simulink model "functional_architecture"  (R2019b)
settings: Solver=VariableStepAuto  StartTime=0.0  StopTime=10.0  RelTol=1e-3
settings Model: Creator=nicol  LastModifiedBy=nicol

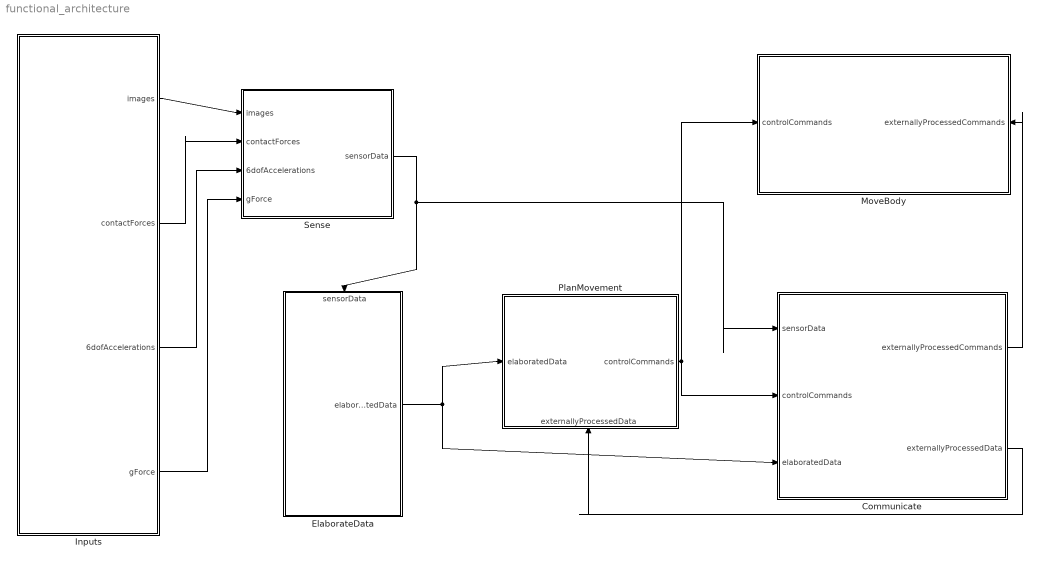
== system functional_architecture ==
  Communicate : Subsystem
      settings: PortSchema="{\"entries\":[{\"content\":{\"headerSize\":26,\"margin\":15,\"minimumSpacing\":25,\"sides\":[{\"content\":{\"connectorIds\":[\"In1\",\"In2\",\"In3\"]},\"type\":\"ConnectorPlacement.EquallySpacedRectSide\",\"uuid\":\"1a5b96a6-6b68-4a44-94ba-f4f30127e72c\"},{\"content\":{\"connectorIds\":[\"Out1\",\"Out2\"],\"side\":\"RIGHT\"},\"type\":\"ConnectorPlacement.EquallySpacedRectSide\",\"uuid\":\"6795999a-37c2-4f74-9b2a-5ff47da3b2b8\"},{\"content\":{\"connectorIds\":[],\"side\":\"TOP\"},\"type\":\"ConnectorPlacement.EquallySpacedRectSide\",\"uuid\":\"71a167ad-2262-404f-8290-656c4c9ef881\"},{\"content\":{\"connectorIds\":[],\"side\":\"BOTTOM\"},\"type\":\"ConnectorPlacement.EquallySpacedRectSide\",\"uuid\":\"bd9bb314-13dd-4e4e-ba5b-ba97c08285c9\"}]},\"type\":\"ConnectorPlacement.EquallySpacedConnector\",\"uuid\":\"f8e426a6-4f1d-49ba-8aa9-835f0600076a\"}],\"packageUris\":[\"http://schema.mathworks.com/mf0/Connector/19700101\"],\"version\":\"1.0\"}"
  ElaborateData : Subsystem
      settings: PortSchema="{\"entries\":[{\"content\":{\"headerSize\":26,\"margin\":15,\"minimumSpacing\":25,\"sides\":[{\"content\":{\"connectorIds\":[]},\"type\":\"ConnectorPlacement.EquallySpacedRectSide\",\"uuid\":\"1a5b96a6-6b68-4a44-94ba-f4f30127e72c\"},{\"content\":{\"connectorIds\":[\"Out1\"],\"side\":\"RIGHT\"},\"type\":\"ConnectorPlacement.EquallySpacedRectSide\",\"uuid\":\"6795999a-37c2-4f74-9b2a-5ff47da3b2b8\"},{\"content\":{\"connectorIds\":[\"In1\"],\"side\":\"TOP\"},\"type\":\"ConnectorPlacement.EquallySpacedRectSide\",\"uuid\":\"71a167ad-2262-404f-8290-656c4c9ef881\"},{\"content\":{\"connectorIds\":[],\"side\":\"BOTTOM\"},\"type\":\"ConnectorPlacement.EquallySpacedRectSide\",\"uuid\":\"ec60985d-ce8e-4674-8cef-feb300bcbcea\"}]},\"type\":\"ConnectorPlacement.EquallySpacedConnector\",\"uuid\":\"f8e426a6-4f1d-49ba-8aa9-835f0600076a\"}],\"packageUris\":[\"http://schema.mathworks.com/mf0/Connector/19700101\"],\"version\":\"1.0\"}"
  Inputs : Subsystem
      settings: PortSchema="{\"entries\":[{\"content\":{\"headerSize\":26,\"margin\":15,\"minimumSpacing\":25,\"sides\":[{\"content\":{\"connectorIds\":[]},\"type\":\"ConnectorPlacement.EquallySpacedRectSide\",\"uuid\":\"1a5b96a6-6b68-4a44-94ba-f4f30127e72c\"},{\"content\":{\"connectorIds\":[\"Out1\",\"Out2\",\"Out3\",\"Out4\"],\"side\":\"RIGHT\"},\"type\":\"ConnectorPlacement.EquallySpacedRectSide\",\"uuid\":\"6795999a-37c2-4f74-9b2a-5ff47da3b2b8\"},{\"content\":{\"connectorIds\":[],\"side\":\"TOP\"},\"type\":\"ConnectorPlacement.EquallySpacedRectSide\",\"uuid\":\"71a167ad-2262-404f-8290-656c4c9ef881\"}]},\"type\":\"ConnectorPlacement.EquallySpacedConnector\",\"uuid\":\"f8e426a6-4f1d-49ba-8aa9-835f0600076a\"}],\"packageUris\":[\"http://schema.mathworks.com/mf0/Connector/19700101\"],\"version\":\"1.0\"}"
  MoveBody : Subsystem
      settings: PortSchema="{\"entries\":[{\"content\":{\"headerSize\":26,\"margin\":15,\"minimumSpacing\":25,\"sides\":[{\"content\":{\"connectorIds\":[\"In2\"]},\"type\":\"ConnectorPlacement.EquallySpacedRectSide\",\"uuid\":\"1a5b96a6-6b68-4a44-94ba-f4f30127e72c\"},{\"content\":{\"connectorIds\":[\"In1\"],\"side\":\"RIGHT\"},\"type\":\"ConnectorPlacement.EquallySpacedRectSide\",\"uuid\":\"6795999a-37c2-4f74-9b2a-5ff47da3b2b8\"},{\"content\":{\"connectorIds\":[],\"side\":\"TOP\"},\"type\":\"ConnectorPlacement.EquallySpacedRectSide\",\"uuid\":\"71a167ad-2262-404f-8290-656c4c9ef881\"},{\"content\":{\"connectorIds\":[],\"side\":\"BOTTOM\"},\"type\":\"ConnectorPlacement.EquallySpacedRectSide\",\"uuid\":\"ac9fe140-66f2-4256-968c-2b10322560fd\"}]},\"type\":\"ConnectorPlacement.EquallySpacedConnector\",\"uuid\":\"f8e426a6-4f1d-49ba-8aa9-835f0600076a\"}],\"packageUris\":[\"http://schema.mathworks.com/mf0/Connector/19700101\"],\"version\":\"1.0\"}"
  PlanMovement : Subsystem
      settings: PortSchema="{\"entries\":[{\"content\":{\"headerSize\":26,\"margin\":15,\"minimumSpacing\":25,\"sides\":[{\"content\":{\"connectorIds\":[\"In1\"]},\"type\":\"ConnectorPlacement.EquallySpacedRectSide\",\"uuid\":\"1a5b96a6-6b68-4a44-94ba-f4f30127e72c\"},{\"content\":{\"connectorIds\":[\"Out1\"],\"side\":\"RIGHT\"},\"type\":\"ConnectorPlacement.EquallySpacedRectSide\",\"uuid\":\"6795999a-37c2-4f74-9b2a-5ff47da3b2b8\"},{\"content\":{\"connectorIds\":[],\"side\":\"TOP\"},\"type\":\"ConnectorPlacement.EquallySpacedRectSide\",\"uuid\":\"71a167ad-2262-404f-8290-656c4c9ef881\"},{\"content\":{\"connectorIds\":[\"In2\"],\"side\":\"BOTTOM\"},\"type\":\"ConnectorPlacement.EquallySpacedRectSide\",\"uuid\":\"7978899b-6d5b-49fc-849e-56f3629990a5\"}]},\"type\":\"ConnectorPlacement.EquallySpacedConnector\",\"uuid\":\"f8e426a6-4f1d-49ba-8aa9-835f0600076a\"}],\"packageUris\":[\"http://schema.mathworks.com/mf0/Connector/19700101\"],\"version\":\"1.0\"}"
  Sense : Subsystem
      settings: PortSchema="{\"entries\":[{\"content\":{\"headerSize\":26,\"margin\":15,\"minimumSpacing\":25,\"sides\":[{\"content\":{\"connectorIds\":[\"In1\",\"In2\",\"In3\",\"In4\"]},\"type\":\"ConnectorPlacement.EquallySpacedRectSide\",\"uuid\":\"1a5b96a6-6b68-4a44-94ba-f4f30127e72c\"},{\"content\":{\"connectorIds\":[\"Out1\"],\"side\":\"RIGHT\"},\"type\":\"ConnectorPlacement.EquallySpacedRectSide\",\"uuid\":\"6795999a-37c2-4f74-9b2a-5ff47da3b2b8\"},{\"content\":{\"connectorIds\":[],\"side\":\"TOP\"},\"type\":\"ConnectorPlacement.EquallySpacedRectSide\",\"uuid\":\"71a167ad-2262-404f-8290-656c4c9ef881\"}]},\"type\":\"ConnectorPlacement.EquallySpacedConnector\",\"uuid\":\"f8e426a6-4f1d-49ba-8aa9-835f0600076a\"}],\"packageUris\":[\"http://schema.mathworks.com/mf0/Connector/19700101\"],\"version\":\"1.0\"}"
  wires:
  Inputs/4(gForce) -> Sense/4(gForce)
  Inputs/3(6dofAccelerations) -> Sense/3(6dofAccelerations)
  Inputs/2(contactForces) -> Sense/2(contactForces)
  Inputs/1(images) -> Sense/1(images)
  Communicate/2(externallyProcessedData) -> PlanMovement/2(externallyProcessedData)
  PlanMovement/1(controlCommands) -> MoveBody/2(controlCommands), Communicate/2(controlCommands)
  ElaborateData/1(elaboratedData) -> Communicate/3(elaboratedData), PlanMovement/1(elaboratedData)
  Sense/1(sensorData) -> Communicate/1(sensorData), ElaborateData/1(sensorData)
  Communicate/1(externallyProcessedCommands) -> MoveBody/1(externallyProcessedCommands)

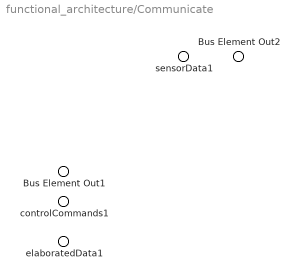
== system functional_architecture/Communicate ==
  sensorData1 : Inport  PortName=sensorData
  controlCommands1 : Inport  Port=2  PortName=controlCommands
  elaboratedData1 : Inport  Port=3  PortName=elaboratedData
  Bus Element Out2 : Outport  PortName=externallyProcessedCommands
  Bus Element Out1 : Outport  Port=2  PortName=externallyProcessedData

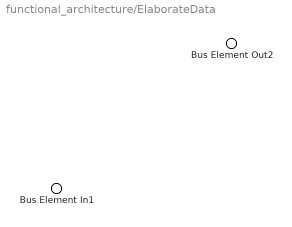
== system functional_architecture/ElaborateData ==
  Bus Element In1 : Inport  PortName=sensorData
  Bus Element Out2 : Outport  PortName=elaboratedData

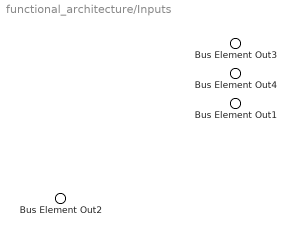
== system functional_architecture/Inputs ==
  Bus Element Out1 : Outport  PortName=images
  Bus Element Out4 : Outport  Port=2  PortName=contactForces
  Bus Element Out3 : Outport  Port=3  PortName=6dofAccelerations
  Bus Element Out2 : Outport  Port=4  PortName=gForce

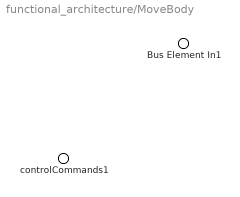
== system functional_architecture/MoveBody ==
  Bus Element In1 : Inport  PortName=externallyProcessedCommands
  controlCommands1 : Inport  Port=2  PortName=controlCommands

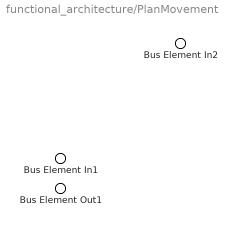
== system functional_architecture/PlanMovement ==
  Bus Element In2 : Inport  PortName=elaboratedData
  Bus Element In1 : Inport  Port=2  PortName=externallyProcessedData
  Bus Element Out1 : Outport  PortName=controlCommands

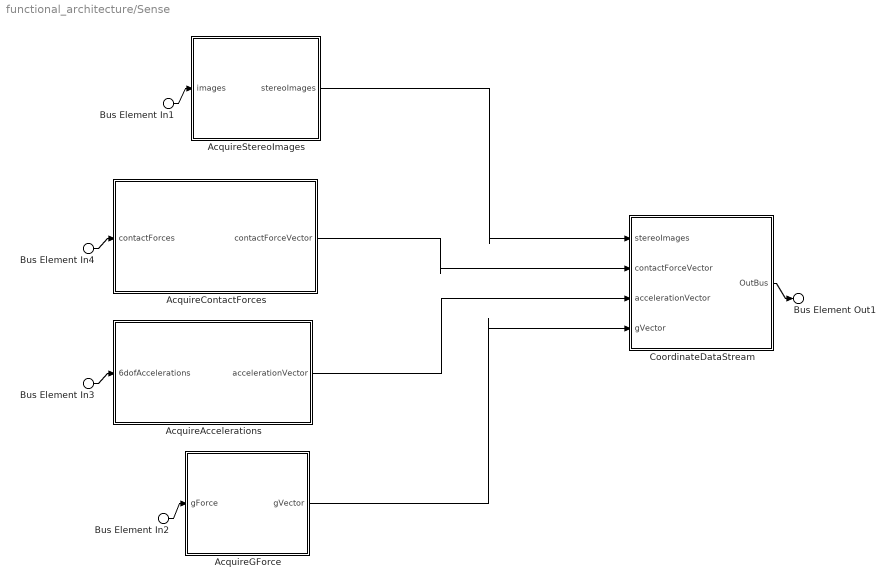
== system functional_architecture/Sense ==
  Bus Element In1 : Inport  PortName=images
  Bus Element In4 : Inport  Port=2  PortName=contactForces
  Bus Element In3 : Inport  Port=3  PortName=6dofAccelerations
  Bus Element In2 : Inport  Port=4  PortName=gForce
  AcquireAccelerations : Subsystem
      settings: PortSchema="{\"entries\":[{\"content\":{\"headerSize\":26,\"margin\":15,\"minimumSpacing\":25,\"sides\":[{\"content\":{\"connectorIds\":[\"In1\"]},\"type\":\"ConnectorPlacement.EquallySpacedRectSide\",\"uuid\":\"1a5b96a6-6b68-4a44-94ba-f4f30127e72c\"},{\"content\":{\"connectorIds\":[\"Out1\"],\"side\":\"RIGHT\"},\"type\":\"ConnectorPlacement.EquallySpacedRectSide\",\"uuid\":\"6795999a-37c2-4f74-9b2a-5ff47da3b2b8\"},{\"content\":{\"connectorIds\":[],\"side\":\"TOP\"},\"type\":\"ConnectorPlacement.EquallySpacedRectSide\",\"uuid\":\"71a167ad-2262-404f-8290-656c4c9ef881\"}]},\"type\":\"ConnectorPlacement.EquallySpacedConnector\",\"uuid\":\"f8e426a6-4f1d-49ba-8aa9-835f0600076a\"}],\"packageUris\":[\"http://schema.mathworks.com/mf0/Connector/19700101\"],\"version\":\"1.0\"}"
  AcquireContactForces : Subsystem
      settings: PortSchema="{\"entries\":[{\"content\":{\"headerSize\":26,\"margin\":15,\"minimumSpacing\":25,\"sides\":[{\"content\":{\"connectorIds\":[\"In1\"]},\"type\":\"ConnectorPlacement.EquallySpacedRectSide\",\"uuid\":\"1a5b96a6-6b68-4a44-94ba-f4f30127e72c\"},{\"content\":{\"connectorIds\":[\"Out1\"],\"side\":\"RIGHT\"},\"type\":\"ConnectorPlacement.EquallySpacedRectSide\",\"uuid\":\"6795999a-37c2-4f74-9b2a-5ff47da3b2b8\"},{\"content\":{\"connectorIds\":[],\"side\":\"TOP\"},\"type\":\"ConnectorPlacement.EquallySpacedRectSide\",\"uuid\":\"71a167ad-2262-404f-8290-656c4c9ef881\"}]},\"type\":\"ConnectorPlacement.EquallySpacedConnector\",\"uuid\":\"f8e426a6-4f1d-49ba-8aa9-835f0600076a\"}],\"packageUris\":[\"http://schema.mathworks.com/mf0/Connector/19700101\"],\"version\":\"1.0\"}"
  AcquireGForce : Subsystem
      settings: PortSchema="{\"entries\":[{\"content\":{\"headerSize\":26,\"margin\":15,\"minimumSpacing\":25,\"sides\":[{\"content\":{\"connectorIds\":[\"In1\"]},\"type\":\"ConnectorPlacement.EquallySpacedRectSide\",\"uuid\":\"1a5b96a6-6b68-4a44-94ba-f4f30127e72c\"},{\"content\":{\"connectorIds\":[\"Out1\"],\"side\":\"RIGHT\"},\"type\":\"ConnectorPlacement.EquallySpacedRectSide\",\"uuid\":\"6795999a-37c2-4f74-9b2a-5ff47da3b2b8\"},{\"content\":{\"connectorIds\":[],\"side\":\"TOP\"},\"type\":\"ConnectorPlacement.EquallySpacedRectSide\",\"uuid\":\"71a167ad-2262-404f-8290-656c4c9ef881\"}]},\"type\":\"ConnectorPlacement.EquallySpacedConnector\",\"uuid\":\"f8e426a6-4f1d-49ba-8aa9-835f0600076a\"}],\"packageUris\":[\"http://schema.mathworks.com/mf0/Connector/19700101\"],\"version\":\"1.0\"}"
  AcquireStereoImages : Subsystem
      settings: PortSchema="{\"entries\":[{\"content\":{\"headerSize\":26,\"margin\":15,\"minimumSpacing\":25,\"sides\":[{\"content\":{\"connectorIds\":[\"In1\"]},\"type\":\"ConnectorPlacement.EquallySpacedRectSide\",\"uuid\":\"1a5b96a6-6b68-4a44-94ba-f4f30127e72c\"},{\"content\":{\"connectorIds\":[\"Out1\"],\"side\":\"RIGHT\"},\"type\":\"ConnectorPlacement.EquallySpacedRectSide\",\"uuid\":\"6795999a-37c2-4f74-9b2a-5ff47da3b2b8\"},{\"content\":{\"connectorIds\":[],\"side\":\"TOP\"},\"type\":\"ConnectorPlacement.EquallySpacedRectSide\",\"uuid\":\"71a167ad-2262-404f-8290-656c4c9ef881\"}]},\"type\":\"ConnectorPlacement.EquallySpacedConnector\",\"uuid\":\"f8e426a6-4f1d-49ba-8aa9-835f0600076a\"}],\"packageUris\":[\"http://schema.mathworks.com/mf0/Connector/19700101\"],\"version\":\"1.0\"}"
  CoordinateDataStream : Subsystem
      settings: PortSchema="{\"entries\":[{\"content\":{\"headerSize\":26,\"margin\":15,\"minimumSpacing\":25,\"sides\":[{\"content\":{\"connectorIds\":[\"In1\",\"In2\",\"In3\",\"In4\"]},\"type\":\"ConnectorPlacement.EquallySpacedRectSide\",\"uuid\":\"1a5b96a6-6b68-4a44-94ba-f4f30127e72c\"},{\"content\":{\"connectorIds\":[\"Out1\"],\"side\":\"RIGHT\"},\"type\":\"ConnectorPlacement.EquallySpacedRectSide\",\"uuid\":\"6795999a-37c2-4f74-9b2a-5ff47da3b2b8\"},{\"content\":{\"connectorIds\":[],\"side\":\"TOP\"},\"type\":\"ConnectorPlacement.EquallySpacedRectSide\",\"uuid\":\"71a167ad-2262-404f-8290-656c4c9ef881\"}]},\"type\":\"ConnectorPlacement.EquallySpacedConnector\",\"uuid\":\"f8e426a6-4f1d-49ba-8aa9-835f0600076a\"}],\"packageUris\":[\"http://schema.mathworks.com/mf0/Connector/19700101\"],\"version\":\"1.0\"}"
  Bus Element Out1 : Outport  PortName=sensorData
  wires:
  Bus Element In1/1 -> AcquireStereoImages/1(images)
  Bus Element In4/1 -> AcquireContactForces/1(contactForces)
  Bus Element In3/1 -> AcquireAccelerations/1(6dofAccelerations)
  Bus Element In2/1 -> AcquireGForce/1(gForce)
  AcquireStereoImages/1(stereoImages) -> CoordinateDataStream/1(stereoImages)
  AcquireContactForces/1(contactForceVector) -> CoordinateDataStream/2(contactForceVector)
  AcquireAccelerations/1(accelerationVector) -> CoordinateDataStream/3(accelerationVector)
  AcquireGForce/1(gVector) -> CoordinateDataStream/4(gVector)
  CoordinateDataStream/1(OutBus) -> Bus Element Out1/1

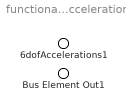
== system functional_architecture/Sense/AcquireAccelerations ==
  6dofAccelerations1 : Inport  PortName=6dofAccelerations
  Bus Element Out1 : Outport  PortName=accelerationVector

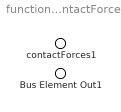
== system functional_architecture/Sense/AcquireContactForces ==
  contactForces1 : Inport  PortName=contactForces
  Bus Element Out1 : Outport  PortName=contactForceVector

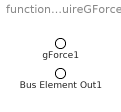
== system functional_architecture/Sense/AcquireGForce ==
  gForce1 : Inport  PortName=gForce
  Bus Element Out1 : Outport  PortName=gVector

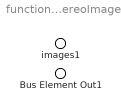
== system functional_architecture/Sense/AcquireStereoImages ==
  images1 : Inport  PortName=images
  Bus Element Out1 : Outport  PortName=stereoImages

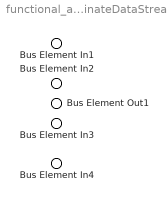
== system functional_architecture/Sense/CoordinateDataStream ==
  Bus Element In1 : Inport  PortName=stereoImages
  Bus Element In2 : Inport  Port=2  PortName=contactForceVector
  Bus Element In3 : Inport  Port=3  PortName=accelerationVector
  Bus Element In4 : Inport  Port=4  PortName=gVector
  Bus Element Out1 : Outport  PortName=OutBus
